simulink model "Main_bikesim"  (R2022b)
settings: Solver=FixedStepAuto  StartTime=0.0  StopTime=sim_time-0.02  FixedStep=0.005
values from neighbouring files (symbols this model uses):
  A_d = (eye(size(A))+Ts*A)    [Kalman_offline.m]    (also in Main_sim.m; Startup_Script.m; Startup_labview.m; Test_ss.m)
  Ad_t = (eye(size(A_t))+Ts*A_t)    [Main_sim.m]    (also in Startup_Script.m; Startup_labview.m)
  B_d = Ts*B    [Kalman_offline.m]    (also in Main_sim.m; Startup_Script.m; Startup_labview.m; Test_ss.m)
  Bd_t = B_t*Ts    [Main_sim.m]    (also in Startup_Script.m; Startup_labview.m)
  bike_model = 1    [Main_sim.m]    (also in Startup_Script.m; Startup_Script_v2.m)
  bike_params = LoadBikeParameters(bike)    [Kalman_offline.m]    (also in Main_sim.m; Startup_Script.m; Startup_Script_v2.m; Startup_labview.m)
  C1 = [1 0 0 0 0 0 0 ... (first row only)    [Kalman_offline.m]    (also in Main_sim.m; Startup_Script.m; Startup_labview.m)
  C2 = [g+((-h_imu*g)/h) 0 (-h_imu*(h*v^2-(g*lr*c)))*sin(lambda)/((lr+lf)*h^2) + (v^2)*sin(lambda)/(lr+lf) 0 ... (first row only)    [Kalman_offline.m]    (also in Main_sim.m = [(-g+((-h_imu*g)/h)) 0 (-h_imu*(h*v^2-(g*lr*c)))*sin(lambda); Startup_Script.m = [(-g+((-h_imu*g)/h)) 0 (-h_imu*(h*v^2-(g*lr*c)))*sin(lambda); Startup_labview.m = [(g+((-h_imu*g)/h)) 0 (-h_imu*(h*v^2-(g*lr*c)))*sin(lambda)/)
  counter = (Ts_GPS / Ts) - 1    (= 9)    [Kalman_offline.m]    (also in Main_sim.m; Startup_Script.m; Startup_labview.m)
  D1 = [0 0 (-h_imu*lr*v)*sin(lambda)/((lr+lf)*h) 0 0 0 0]'    [Kalman_offline.m]    (also in Main_sim.m = [0 0 (-h_imu*lr*v)/((lr+lf)*h) 0 0 0 0]'; Startup_Script.m = [0 0 (-h_imu*lr*v)/((lr+lf)*h) 0 0 0 0]'; Startup_labview.m = [0 0 (-h_imu*lr*v)/((lr+lf)*h) 0 0 0 0]')
  D2 = [(-h_imu*lr*v)*sin(lambda)/((lr+lf)*h) 0 0 0 0]'    [Kalman_offline.m]    (also in Main_sim.m = [(-h_imu*lr*v)/((lr+lf)*h) 0 0 0 0]'; Startup_Script.m = [(-h_imu*lr*v)/((lr+lf)*h) 0 0 0 0]'; Startup_labview.m = [(-h_imu*lr*v)/((lr+lf)*h) 0 0 0 0]')
  e1_max = abs(-k2*e2_max/k1)    [Main_sim.m]    (also in Startup_Script.m; Startup_Script_v2.m; Startup_labview.m)
  g = -9.81    [Kalman_offline.m]    (also in Main_sim.m = 9.81; Startup_Script.m = 9.81; Startup_Script_v2.m = 9.81; Startup_labview.m = 9.81)
  hor_dis = 10    [Main_sim.m]    (also in Startup_Script.m = 1; Startup_Script_v2.m = 1)
  I_balancing_outer = 0.0    (= 0)    [Main_sim.m]    (also in Startup_Script.m; Startup_Script_v2.m; Startup_labview.m)
  initial_state_estimate = initial_state    [Main_sim.m]    (also in Startup_Script.m; Startup_Script_v2.m)
  k1 = K(1)    [Main_sim.m]    (also in Startup_Script.m; Startup_Script_v2.m; Startup_labview.m)
  k2 = K(2)    [Main_sim.m]    (also in Startup_Script.m; Startup_Script_v2.m; Startup_labview.m)
  Kalman_gain1 = Kalman_gain1'    [Kalman_offline.m]    (also in Main_sim.m; Startup_Script.m; Startup_labview.m)
  Kalman_gain2 = Kalman_gain2'    [Kalman_offline.m]    (also in Main_sim.m = Kalman_gain1(4:7,3:7); Startup_Script.m = Kalman_gain1(4:7,3:7); Startup_labview.m = Kalman_gain1(4:7,3:7))
  linearized_sys = ss(A,B,C,D)    [Startup_Script_v2.m]
  P_balancing_inner = 3    [Main_sim.m]    (also in Startup_Script.m = 1; Startup_Script_v2.m; Startup_labview.m = 1)
  P_balancing_outer = 1.3    [Main_sim.m]    (also in Startup_Script.m = 1.75; Startup_Script_v2.m; Startup_labview.m = 1.75)
  Psiref = psiref'    [ReferenceGenerator.m]
  ref_dis = 0.01    [Main_sim.m]    (also in Startup_Script.m; Startup_Script_v2.m = 0.22)
  ref_start_idx = 2    [Main_sim.m]    (also in Startup_Script.m)
  T = Rz*Ry*Rx    [Main_sim.m]    (also in Startup_Script.m)
  Ts = 0.01    [Kalman_offline.m]    (also in Main_sim.m; Startup_Script.m; Startup_Script_v2.m; Startup_labview.m)
  v = 3    [Main_sim.m]    (also in Startup_Script.m = 2; Startup_Script_v2.m; Startup_labview.m = 2; Test_ss.m)
  Xref = xref'    [ReferenceGenerator.m]
  Yref = yref'    [ReferenceGenerator.m]
undefined symbols (not defined in the file or in its folder): C_t, D_t, initial_state, pert_deltadot_state, pert_deltadot_state_fun, pert_phidot_state, pert_phidot_state_fun, sigbuilder_block
libraries: simulink x8, slpidlib x2, eeGeneralControl x1
(part 2 of 2)

== matlab function Main_bikesim/State estimator1/Linearized Bicycle Model on Constant Velocity ==
  data: Est_States input; dot_delta input; y input; Kalman_gain1 input; Kalman_gain2 input; bike_params input; Est_states output; flag input; A_d parameter; B_d parameter; C1 parameter; C2 parameter; D1 parameter; D2 parameter; T parameter
function Est_states  = fcn(Est_States, dot_delta, y, Kalman_gain1, Kalman_gain2, bike_params, flag, A_d, B_d, C1, C2, D1, D2, T)
% description 
% Inputs
%   Est_States := [X Y psi phi phi_dot delta v] are global at time t 
%   dot_delta_e := effective steering rate
%   y := measurement vector
%   Kalman_gain1 := Computed state_feedback gain including GPS meas
%   Kalman_gain2 := Computed state_feedback gain excluding GPS meas
%   bike_params := vector of bike parameters + gravity
%   Ts := Estimator sampling rate
%   v := constant velocity
%   flag := [0-1] increasing counter reseted at 1. When flag == 0 means
%           that GPS measurement is available
%
% Outputs
%   Est_states : = [X Y psi phi phi_dot delta v] global at time t+1


% Transform the states to local frame 
    Est_States_l = zeros(7,1);
    
    Est_States_l(1) = Est_States(1) * cos(Est_States(3)) + Est_States(2) * sin(Est_States(3));
    Est_States_l(2) = -Est_States(1) * sin(Est_States(3)) + Est_States(2) * cos(Est_States(3));
    Est_States_l(3) = 0;        % direction of bike is aligned with X local frame
    Est_States_l(4) = Est_States(4);
    Est_States_l(5) = Est_States(5);
    Est_States_l(6) = Est_States(6);
    Est_States_l(7) = Est_States(7);

% Transform measurements to local frame
    y_l = zeros(size(y));

    y_l(1) = y(1) * cos(Est_States(3)) + y(2) * sin(Est_States(3));
    y_l(2) = -y(1) * sin(Est_States(3)) + y(2) * cos(Est_States(3)); 
    y_l(3) = y(3);
    y_l(4) = y(4);
    y_l(5) = y(5);
    y_l(6) = y(6);
    y_l(7) = y(7);

% Correct for parameter values/sensor positions
% The parameters/positions are measures by us (can differ from true values)
X_gps_mod = bike_params(1);
Y_gps_mod = bike_params(2);
H_gps_mod = bike_params(3);

y_l(1) = y_l(1) - X_gps_mod;
y_l(2) = y_l(2) - Y_gps_mod - H_gps_mod*sin(Est_States(4));

% IMU correction
raw_acc  = [0 y_l(3) 0];
raw_gyro = [y_l(4) 0 y_l(5)];

% Apply the correction to the accelerometer measurement
acc_corr = T*raw_acc';

% Apply the correction to the gyro measurement
gyro_corr = T*raw_gyro';
% Results
y_l(3) =acc_corr(2) ;
y_l(4) =gyro_corr(1) ;
y_l(5) =gyro_corr(3) ;
% 
% % Continuous Time update in local frame TODO: x(t+1) = (I+A delta_T)h_hat(t)
%     states_dot = zeros(7,1);
%     
%     states_dot(1) = Est_States(7);
%     states_dot(2) = v * (Est_States_l(3) + (lr/(lr+lf))*Est_States(6) );
%     states_dot(3) = (v/(lr+lf)) * Est_States(6);
%     states_dot(4) = Est_States(5);
%     states_dot(5) =(g/h)*Est_States(4) + ((lr*v)/((lr+lf)*h))*sin(lambda)*dot_delta + ((h*v^2-g*lr*c)/((lr+lf)*h^2))*sin(lambda)*Est_States(6);
%     states_dot(6) = dot_delta;
%     states_dot(7) = 0;
% 
% % Discrete time update in local 
%     Est_States_l = Est_States_l + states_dot * Ts; 

% % C identity is used to see if the code runs
%     sen = zeros(6,1);
%     sen(1)      = States_l(1);  
%     sen(2)      = States_l(2);
%     %sen(3)      = States_l(3);
%     sen(3)      = States_l(4);
%     sen(4)      = States_l(5);
%     sen(5)      = States_l(6);
%     sen(6)      = States_l(7);

% % Transform measurements into local frame to see if code runs
%     meas_l = zeros(6,1);
%     meas_l(1) = meas(1) * cos(States(3)) + meas(2) * sin(States(3));
%     meas_l(2) = -meas(1) * sin(States(3)) + meas(2) * cos(States(3));
%     meas_l(3) = 0;
%     meas_l(3) = meas(3)-States(3);  
%     meas_l(3) = meas(4);
%     meas_l(4) = meas(5);
%     meas_l(5) = meas(6);
%     meas_l(6) = meas(7);
%     meas_l(7) = meas(7);

% Time update in local frame (from t to t+1)

    % Time update
     Est_States_l = A_d*Est_States_l + B_d*dot_delta;

    % Measurement update in local frame
     Est_states_l = zeros(7,1);

    % Sampling differentiation (Sensors rate 100Hz but GPS 10Hz)

    if flag == 0 % GPS sensors included
    
        % Select Kalman Gain
            K = Kalman_gain1;

        % Measurement prediction
            y_pred = C1*Est_States_l + D1*dot_delta;
    
        % Measurement update
            Est_states_l = Est_States_l + K * (y_l - y_pred);
        
    else % GPS sensors excluded
    
        % Select Kalman Gain
            K = Kalman_gain2;
    
        % Measurement prediction
            y_pred = C2*Est_States_l(4:7) + D2*dot_delta;
 
        % Measurement update
        Est_states_l(1) = Est_States_l(1);
        Est_states_l(2) = Est_States_l(2);
        Est_states_l(3) = Est_States_l(3);
%         Est_states_l(4) = Est_States_l(4);
%         Est_states_l(5) = Est_States_l(5);
%         Est_states_l(6) = Est_States_l(6);
%         Est_states_l(7) = Est_States_l(7);
        Est_states_l(4:7) = Est_States_l(4:7) + K * (y_l(3:7) - y_pred);

    end

    % states_l = Kalman_gain * (meas_l - sen);
    % states_l(1) = States_l(1) + Kalman_gain(1,1) * (meas_l(1) - x_m) + Kalman_gain(1,2) * (meas_l(2) - y_m) + Kalman_gain(1,3) * (meas_l(3) - psi_m) + Kalman_gain(1,4) * (meas_l(4) - phi_m) + Kalman_gain(1,5) * (meas_l(5) - dot_phi_m) + Kalman_gain(1,6) * (meas_l(6) - delta_m) + Kalman_gain(1,7) * (meas_l(7) - v_m);
    % states_l(2) = States_l(2) + Kalman_gain(2,1) * (meas_l(1) - x_m) + Kalman_gain(2,2) * (meas_l(2) - y_m) + Kalman_gain(2,3) * (meas_l(3) - psi_m) + Kalman_gain(2,4) * (meas_l(4) - phi_m) + Kalman_gain(2,5) * (meas_l(5) - dot_phi_m) + Kalman_gain(2,6) * (meas_l(6) - delta_m) + Kalman_gain(2,7) * (meas_l(7) - v_m);
    % states_l(3) = States_l(3) + Kalman_gain(3,1) * (meas_l(1) - x_m) + Kalman_gain(3,2) * (meas_l(2) - y_m) + Kalman_gain(3,3) * (meas_l(3) - psi_m) + Kalman_gain(3,4) * (meas_l(4) - phi_m) + Kalman_gain(3,5) * (meas_l(5) - dot_phi_m) + Kalman_gain(3,6) * (meas_l(6) - delta_m) + Kalman_gain(3,7) * (meas_l(7) - v_m);
    % states_l(4) = States_l(4) + Kalman_gain(4,1) * (meas_l(1) - x_m) + Kalman_gain(4,2) * (meas_l(2) - y_m) + Kalman_gain(4,3) * (meas_l(3) - psi_m) + Kalman_gain(4,4) * (meas_l(4) - phi_m) + Kalman_gain(4,5) * (meas_l(5) - dot_phi_m) + Kalman_gain(4,6) * (meas_l(6) - delta_m) + Kalman_gain(4,7) * (meas_l(7) - v_m);
    % states_l(5) = States_l(5) + Kalman_gain(5,1) * (meas_l(1) - x_m) + Kalman_gain(5,2) * (meas_l(2) - y_m) + Kalman_gain(5,3) * (meas_l(3) - psi_m) + Kalman_gain(5,4) * (meas_l(4) - phi_m) + Kalman_gain(5,5) * (meas_l(5) - dot_phi_m) + Kalman_gain(5,6) * (meas_l(6) - delta_m) + Kalman_gain(5,7) * (meas_l(7) - v_m);
    % states_l(6) = States_l(6) + Kalman_gain(6,1) * (meas_l(1) - x_m) + Kalman_gain(6,2) * (meas_l(2) - y_m) + Kalman_gain(6,3) * (meas_l(3) - psi_m) + Kalman_gain(6,4) * (meas_l(4) - phi_m) + Kalman_gain(6,5) * (meas_l(5) - dot_phi_m) + Kalman_gain(6,6) * (meas_l(6) - delta_m) + Kalman_gain(6,7) * (meas_l(7) - v_m);
    % states_l(7) = States_l(7) + Kalman_gain(7,1) * (meas_l(1) - x_m) + Kalman_gain(7,2) * (meas_l(2) - y_m) + Kalman_gain(7,3) * (meas_l(3) - psi_m) + Kalman_gain(7,4) * (meas_l(4) - phi_m) + Kalman_gain(7,5) * (meas_l(5) - dot_phi_m) + Kalman_gain(7,6) * (meas_l(6) - delta_m) + Kalman_gain(7,7) * (meas_l(7) - v_m);

% Transform to global the local states at time t+1 after measurement update
    Est_states = zeros(7,1);
    Est_states(3) = Est_States(3) + Est_states_l(3);    % direction update global
    
    % Change of Coordinates from local to global frame for  states 
    Est_states(1) = Est_states_l(1) * cos(Est_States(3)) - Est_states_l(2) * sin(Est_States(3));
    Est_states(2) = Est_states_l(1) * sin(Est_States(3)) + Est_states_l(2) * cos(Est_States(3));
    Est_states(4) = Est_states_l(4);
    Est_states(5) = Est_states_l(5);
    Est_states(6) = Est_states_l(6);
    Est_states(7) = Est_states_l(7);
    
    % Heading angle between pi and -pi
    Est_states(3) = wrapToPi(Est_states(3));

end

== matlab function Main_bikesim/Unstable bike model1/Nonlinear Bicycle model/MATLAB Function ==
  data: States input; xdot output; Steering_rate input; Speed input; disturbances input; bike_params input
function xdot  = fcn(States, Steering_rate, Speed, disturbances, bike_params)
% Unpacked bike_params
    g = bike_params(1);
    h = bike_params(2);
    lr = bike_params(3);
    lf = bike_params(4);
    lambda = bike_params(5);
    c = bike_params(6);
    m = bike_params(7);
    h_imu = bike_params(8);

phi =   States(1);%roll
delta = States(2);%steering angle
phi_d = States(3);%rollrate

% xdot = [phidot deltadot phiddot]
xdot1 = phi_d + disturbances(1);
xdot2 = Steering_rate + disturbances(2);
xdot3 = (g/h)*sin(phi) + ((lr*Speed)/((lr+lf)*h))/(cos(sin(lambda)*delta)^2)*sin(lambda)*Steering_rate ...
                                  + ((h*Speed^2-g*lr*c)/((lr+lf)*h^2))*sin(lambda)*tan(delta);

% linearized
% xdot3 = (g/h)*phi + ((lr*Speed)/((lr+lf)*h))*Steering_rate + ((h*Speed^2-g*lr*c)/((lr+lf)*h^2))*sin(lambda)*delta;

xdot = [xdot1 xdot2 xdot3]';
